simulink model "LP8"  (R2019a)
settings: Solver=FixedStepDiscrete  StartTime=0.0  StopTime=stop_time  RelTol=1e-3
InitFcn:
  | sm_callback_init
StopFcn:
  | sm_callback_stop
undefined symbols (not defined in the file or in its folder): mp
libraries: simulink x3
settings Model: Creator=Ross  LastModifiedBy=Ross
settings DataIOCC: ReturnWorkspaceOutputs=off
settings OptimizationCC: BlockReduction=off  ConditionallyExecuteInputs=off  DefaultParameterBehavior=Inlined
settings DebuggingCC: ReadBeforeWriteMsg=DisableAll  WriteAfterWriteMsg=DisableAll  WriteAfterReadMsg=DisableAll  AlgebraicLoopMsg=error  MultiTaskDSMMsg=none  SingleTaskRateTransMsg=error  PregeneratedLibrarySubsystemCodeDiagnostic=none  ArithmeticOperatorsInVariantConditions=warning
settings HardwareCC: ProdBitPerPointer=32  ProdBitPerSizeT=32  ProdBitPerPtrDiffT=32  ProdLargestAtomicFloat=None  ProdIntDivRoundTo=Undefined  ProdEndianess=Unspecified  ProdWordSize=32  ProdHWDeviceType=ASIC/FPGA->ASIC/FPGA  TargetBitPerPointer=64  TargetBitPerSizeT=64  TargetBitPerPtrDiffT=64  TargetLongLongMode=on  TargetIntDivRoundTo=Zero  TargetEndianess=LittleEndian  TargetWordSize=64  TargetHWDeviceType=Custom Processor->MATLAB Host Computer  ProdEqTarget=off
settings ModelReferenceCC: UpdateModelReferenceTargets=IfOutOfDate
settings SFSimCC: SFSimEcho=off  SimUseLocalCustomCode=off
settings RTWCC: RTWUseLocalCustomCode=off

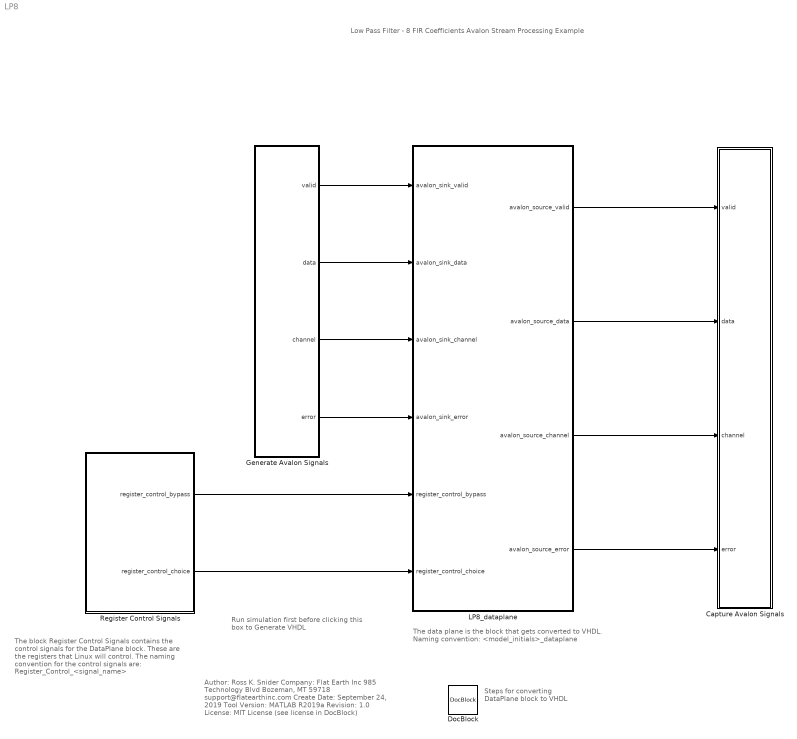
== system LP8 ==
  note: The data plane is the block that gets converted to VHDL. Naming convention: <model_initials>_dataplane
  note: Author:          Ross K. Snider
      | Company:     Flat Earth Inc
      |                       985 Technology Blvd
      |                       Bozeman, MT 59718
      |                       support@flatearthinc.com
      | Create Date:  September 24, 2019
      | Tool Version:  MATLAB R2019a
      | Revision:        1.0
      | License:          MIT License (see license in DocBlock)
  note: Steps for converting
      | DataPlane block
      | to VHDL
  note: Low Pass Filter - 8 FIR Coefficients
      | Avalon Stream Processing Example
  note: Run simulation first
      | before clicking this box to
      | Generate VHDL
  note: The block Register Control Signals contains
      | the control signals for the DataPlane block.
      | These are the registers that Linux will control.
      | The naming convention for the control
      | signals are:  Register_Control_<signal_name>
  Capture Avalon Signals : Subsystem
  DocBlock : simulink/Model-Wide Utilities/DocBlock  DocumentType=HTML
  Generate Avalon Signals : Subsystem
  LP8_dataplane : Subsystem  TreatAsAtomicUnit=on
  Register Control Signals : Subsystem
  wires:
  Generate Avalon Signals/2(data) -> LP8_dataplane/2(avalon_sink_data)
  Generate Avalon Signals/1(valid) -> LP8_dataplane/1(avalon_sink_valid)
  Generate Avalon Signals/3(channel) -> LP8_dataplane/3(avalon_sink_channel)
  Generate Avalon Signals/4(error) -> LP8_dataplane/4(avalon_sink_error)
  LP8_dataplane/2(avalon_source_data) -> Capture Avalon Signals/2(data)
  LP8_dataplane/1(avalon_source_valid) -> Capture Avalon Signals/1(valid)
  LP8_dataplane/3(avalon_source_channel) -> Capture Avalon Signals/3(channel)
  LP8_dataplane/4(avalon_source_error) -> Capture Avalon Signals/4(error)
  Register Control Signals/2(register_control_choice) -> LP8_dataplane/6(register_control_choice)
  Register Control Signals/1(register_control_bypass) -> LP8_dataplane/5(register_control_bypass)

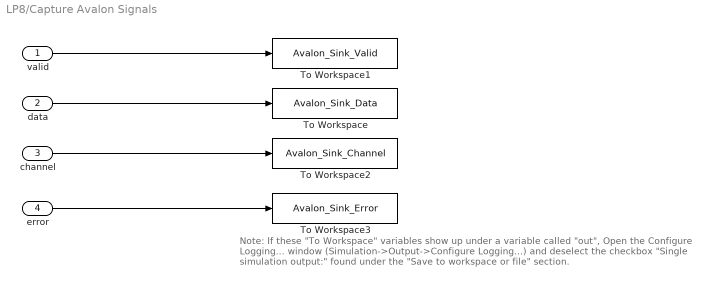
== system LP8/Capture Avalon Signals ==
  note: Note:  If these "To Workspace" variables show up under a variable called "out",
      | Open the Configure Logging... window (Simulation->Output->Configure Logging...)
      | and deselect the checkbox "Single simulation output:" found under the "Save to workspace or file" section.
  valid : Inport
  data : Inport  Port=2
  channel : Inport  Port=3
  error : Inport  Port=4
  To Workspace : ToWorkspace  VariableName=Avalon_Sink_Data  SaveFormat=Timeseries  SampleTime=-1
  To Workspace1 : ToWorkspace  VariableName=Avalon_Sink_Valid  SaveFormat=Timeseries  SampleTime=-1
  To Workspace2 : ToWorkspace  VariableName=Avalon_Sink_Channel  SaveFormat=Timeseries  SampleTime=-1
  To Workspace3 : ToWorkspace  VariableName=Avalon_Sink_Error  SaveFormat=Timeseries  SampleTime=-1
  wires:
  data/1 -> To Workspace/1
  valid/1 -> To Workspace1/1
  error/1 -> To Workspace3/1
  channel/1 -> To Workspace2/1

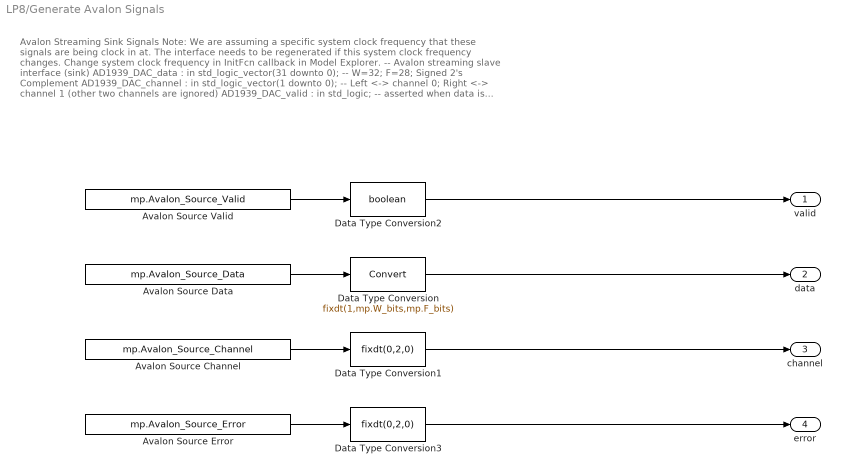
== system LP8/Generate Avalon Signals ==
  note: Avalon Streaming Sink Signals
      | Note: We are assuming a specific system clock frequency that these signals are being clock in at.
      | The interface needs to be regenerated if this system clock frequency changes. Change system clock frequency in InitFcn callback in Model Explorer.
      |
      | -- Avalon streaming slave interface (sink)
      | AD1939_DAC_data : in std_logic_vector(31 downto 0); -- W=32; F=28; Signed 2's Complement
      | AD1939_DAC_channel : in std_logic_vector(1 downto 0); -- Left <-> channel 0; Right <-> channel 1 (other two channels are ignored)
      | AD1939_DAC_valid : in std_logic; -- asserted when data is valid
      | AD1939_DAC_error : in std_logic_vector(1 downto 0) -- error channel is ignored, assumed to be error free at this point
      |
      | For more information on the data-channel-valid protocol, s ee chapter 5 in Intel's Avalon Interfaced Specification (p. 40) at https://www.intel.com/content/dam/www/programmable/us/en/pdfs/literature/manual/mnl_avalon_spec.pdf
  Avalon Source Channel : FromWorkspace  VariableName=mp.Avalon_Source_Channel  OutDataTypeStr=double  SampleTime=mp.Ts_system
  "Avalon Source Data " : FromWorkspace  VariableName=mp.Avalon_Source_Data  OutDataTypeStr=double  SampleTime=mp.Ts_system
  Avalon Source Error : FromWorkspace  VariableName=mp.Avalon_Source_Error  OutDataTypeStr=double  SampleTime=mp.Ts_system
  Avalon Source Valid : FromWorkspace  VariableName=mp.Avalon_Source_Valid  OutDataTypeStr=double  SampleTime=mp.Ts_system
  Data Type Conversion : DataTypeConversion  OutDataTypeStr=fixdt(1,mp.W_bits,mp.F_bits)
  Data Type Conversion1 : DataTypeConversion  OutDataTypeStr=fixdt(0,2,0)
  Data Type Conversion2 : DataTypeConversion  OutDataTypeStr=boolean
  Data Type Conversion3 : DataTypeConversion  OutDataTypeStr=fixdt(0,2,0)
  valid : Outport
  data : Outport  Port=2
  channel : Outport  Port=3
  error : Outport  Port=4
  wires:
  Data Type Conversion1/1 -> channel/1
  Data Type Conversion2/1 -> valid/1
  Avalon Source Error/1 -> Data Type Conversion3/1
  Data Type Conversion/1 -> data/1
  Avalon Source Valid/1 -> Data Type Conversion2/1
  Data Type Conversion3/1 -> error/1
  Avalon Source Channel/1 -> Data Type Conversion1/1
  "Avalon Source Data "/1 -> Data Type Conversion/1

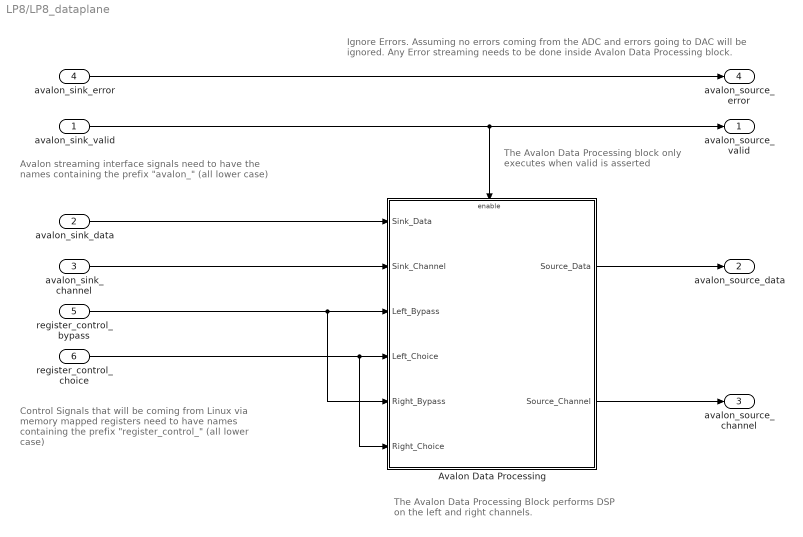
== system LP8/LP8_dataplane ==
  note: Control Signals that will be coming from Linux via
      | memory mapped registers need to have names
      | containing the prefix "register_control_"
      | (all lower case)
  note: The Avalon Data Processing Block
      | performs DSP on the left and right channels.
  note: The Avalon Data Processing block
      | only executes when valid is asserted
  note: Ignore Errors.
      | Assuming no errors coming from the ADC and errors going to DAC will be ignored.
      | Any Error streaming needs to be done inside Avalon Data Processing block.
  note: Avalon streaming interface signals need to have the
      | names containing the prefix "avalon_"
      | (all lower case)
  avalon_sink_valid : Inport
  avalon_sink_data : Inport  Port=2
  avalon_sink_channel : Inport  Port=3
  avalon_sink_error : Inport  Port=4
  register_control_bypass : Inport  Port=5
  register_control_choice : Inport  Port=6
  Avalon Data Processing : Subsystem  TreatAsAtomicUnit=on
  avalon_source_valid : Outport
  avalon_source_data : Outport  Port=2
  avalon_source_channel : Outport  Port=3
  avalon_source_error : Outport  Port=4
  wires:
  avalon_sink_channel/1 -> Avalon Data Processing/2(Sink_Channel)
  avalon_sink_error/1 -> avalon_source_error/1
  Avalon Data Processing/1(Source_Data) -> avalon_source_data/1
  avalon_sink_valid/1 -> avalon_source_valid/1, Avalon Data Processing/Enable
  avalon_sink_data/1 -> Avalon Data Processing/1(Sink_Data)
  Avalon Data Processing/2(Source_Channel) -> avalon_source_channel/1
  register_control_bypass/1 -> Avalon Data Processing/5(Right_Bypass), Avalon Data Processing/3(Left_Bypass)
  register_control_choice/1 -> Avalon Data Processing/6(Right_Choice), Avalon Data Processing/4(Left_Choice)

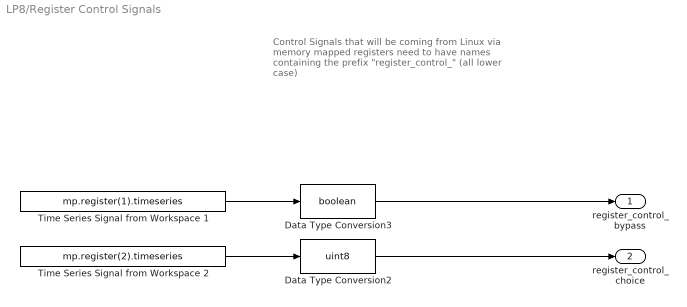
== system LP8/Register Control Signals ==
  note: Control Signals that will be coming from Linux via
      | memory mapped registers need to have names
      | containing the prefix "register_control_"
      | (all lower case)
  Data Type Conversion2 : DataTypeConversion  OutDataTypeStr=uint8
  Data Type Conversion3 : DataTypeConversion  OutDataTypeStr=boolean
  Time Series Signal from Workspace 1 : FromWorkspace  VariableName=mp.register(1).timeseries  OutDataTypeStr=double  SampleTime=mp.Ts_system
  Time Series Signal from Workspace 2 : FromWorkspace  VariableName=mp.register(2).timeseries  OutDataTypeStr=double  SampleTime=mp.Ts_system
  register_control_bypass : Outport
  register_control_choice : Outport  Port=2
  wires:
  Time Series Signal from Workspace 2/1 -> Data Type Conversion2/1
  Data Type Conversion2/1 -> register_control_choice/1
  Time Series Signal from Workspace 1/1 -> Data Type Conversion3/1
  Data Type Conversion3/1 -> register_control_bypass/1

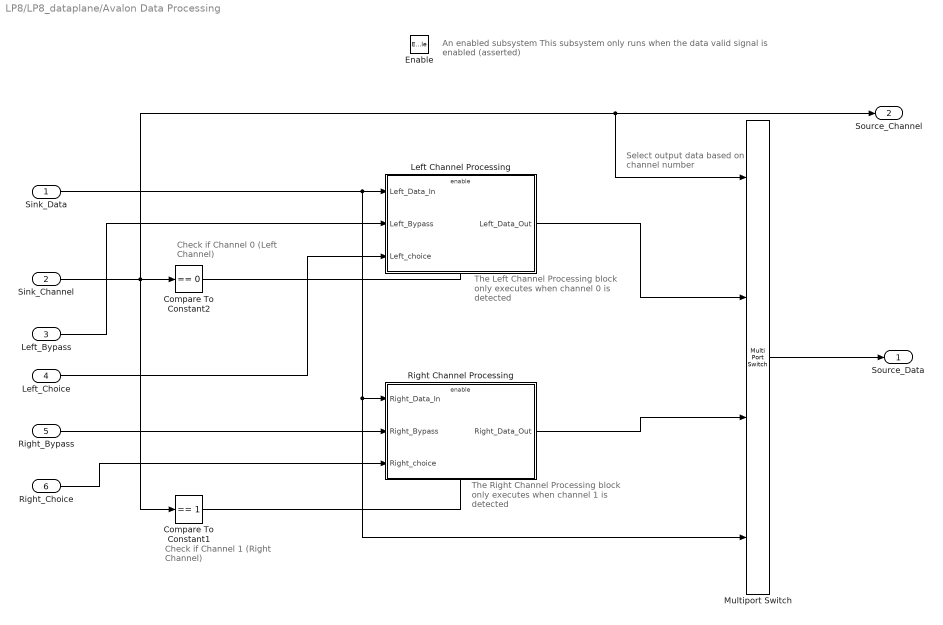
== system LP8/LP8_dataplane/Avalon Data Processing ==
  note: Select output data
      | based on channel number
  note: Check if Channel 0
      | (Left Channel)
  note: The Left Channel Processing block
      | only executes when channel 0
      | is detected
  note: The Right Channel Processing block
      | only executes when channel 1
      | is detected
  note: Check if Channel 1
      | (Right Channel)
  note: An enabled subsystem
      | This subsystem only runs when the data valid signal is enabled (asserted)
  Sink_Data : Inport
  Sink_Channel : Inport  Port=2
  Left_Bypass : Inport  Port=3
  Left_Choice : Inport  Port=4
  Right_Bypass : Inport  Port=5
  Right_Choice : Inport  Port=6
  Enable : EnablePort
  Compare To Constant1 : simulink/Logic and Bit Operations/Compare To Constant  relop===  const=1  OutDataTypeStr=boolean
  Compare To Constant2 : simulink/Logic and Bit Operations/Compare To Constant  relop===  const=0  OutDataTypeStr=boolean
  Left Channel Processing : Subsystem  TreatAsAtomicUnit=on
  Multiport Switch : MultiPortSwitch  DataPortOrder=Zero-based contiguous  zeroidx=on
  Right Channel Processing : Subsystem  TreatAsAtomicUnit=on
  Source_Data : Outport  InitialOutput=0
  Source_Channel : Outport  Port=2  InitialOutput=0
  wires:
  Sink_Channel/1 -> Source_Channel/1, Multiport Switch/1, Compare To Constant1/1, Compare To Constant2/1
  Compare To Constant2/1 -> Left Channel Processing/Enable
  Compare To Constant1/1 -> Right Channel Processing/Enable
  Sink_Data/1 -> Multiport Switch/4, Right Channel Processing/1(Right_Data_In), Left Channel Processing/1(Left_Data_In)
  Left Channel Processing/1("Left_Data_Out ") -> Multiport Switch/2
  Right Channel Processing/1("Right_Data_Out ") -> Multiport Switch/3
  Multiport Switch/1 -> Source_Data/1
  Left_Bypass/1 -> Left Channel Processing/2(Left_Bypass)
  Right_Bypass/1 -> Right Channel Processing/2(Right_Bypass)
  Left_Choice/1 -> Left Channel Processing/3(Left_choice)
  Right_Choice/1 -> Right Channel Processing/3(Right_choice)

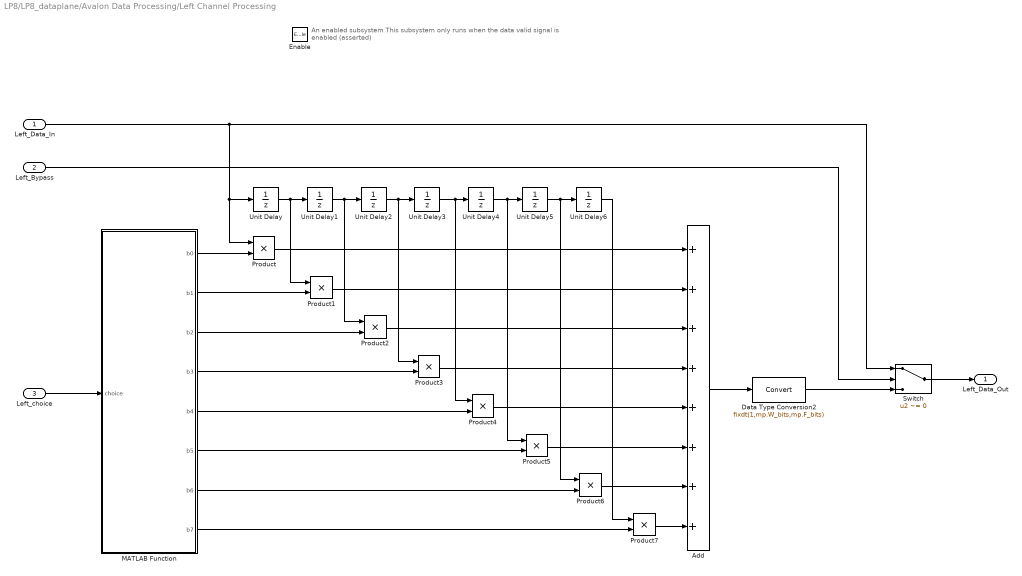
== system LP8/LP8_dataplane/Avalon Data Processing/Left Channel Processing ==
  note: An enabled subsystem
      | This subsystem only runs when the data valid signal is enabled (asserted)
  Left_Data_In : Inport
  Left_Bypass : Inport  Port=2
  Left_choice : Inport  Port=3
  Enable : EnablePort
  Add : Sum  Inputs=++++++++
  Data Type Conversion2 : DataTypeConversion  OutDataTypeStr=fixdt(1,mp.W_bits,mp.F_bits)
  MATLAB Function : MATLAB Function  TreatAsAtomicUnit=on
  Product{,1..7} (8 alike) : Product
  Switch : Switch  Criteria=u2 ~= 0
  Unit Delay{,1..6} (7 alike) : UnitDelay  SampleTime=-1  HasFrameUpgradeWarning=on
  "Left_Data_Out " : Outport  InitialOutput=0
  wires:
  Left_Data_In/1 -> Product/1, Unit Delay/1, Switch/1
  Data Type Conversion2/1 -> Switch/3
  Switch/1 -> "Left_Data_Out "/1
  Left_Bypass/1 -> Switch/2
  Unit Delay/1 -> Product1/1, Unit Delay1/1
  Unit Delay1/1 -> Product2/1, Unit Delay2/1
  Unit Delay2/1 -> Product3/1, Unit Delay3/1
  Unit Delay3/1 -> Product4/1, Unit Delay4/1
  Unit Delay4/1 -> Product5/1, Unit Delay5/1
  Unit Delay5/1 -> Product6/1, Unit Delay6/1
  Unit Delay6/1 -> Product7/1
  Product/1 -> Add/1
  Product1/1 -> Add/2
  Product2/1 -> Add/3
  Product3/1 -> Add/4
  Product4/1 -> Add/5
  Product5/1 -> Add/6
  Product6/1 -> Add/7
  Product7/1 -> Add/8
  Add/1 -> Data Type Conversion2/1
  MATLAB Function/1(b0) -> Product/2
  MATLAB Function/8(b7) -> Product7/2
  MATLAB Function/2(b1) -> Product1/2
  MATLAB Function/3(b2) -> Product2/2
  MATLAB Function/4(b3) -> Product3/2
  MATLAB Function/5(b4) -> Product4/2
  MATLAB Function/6(b5) -> Product5/2
  MATLAB Function/7(b6) -> Product6/2
  Left_choice/1 -> MATLAB Function/1(choice)

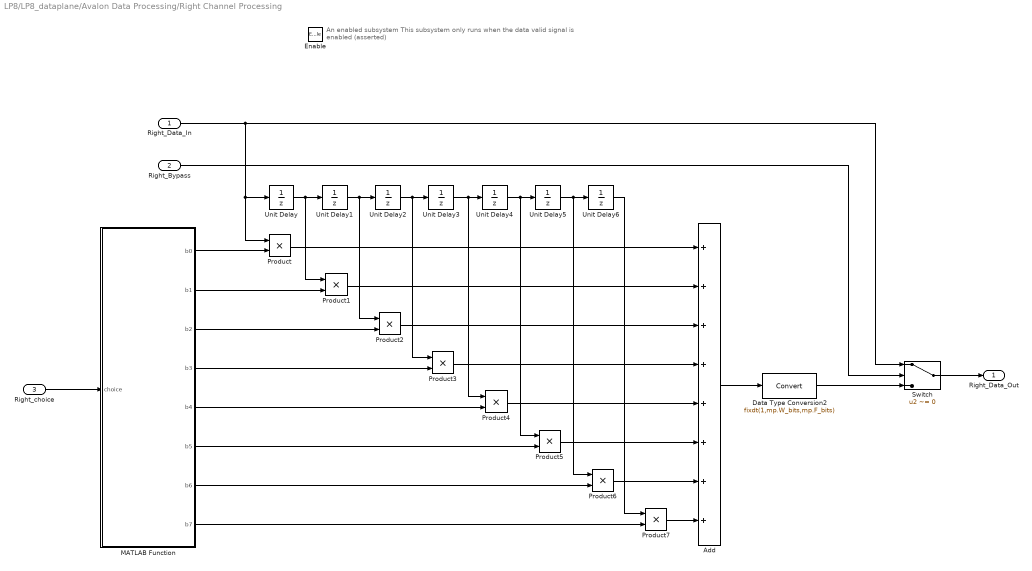
== system LP8/LP8_dataplane/Avalon Data Processing/Right Channel Processing ==
  note: An enabled subsystem
      | This subsystem only runs when the data valid signal is enabled (asserted)
  Right_Data_In : Inport
  Right_Bypass : Inport  Port=2
  Right_choice : Inport  Port=3
  Enable : EnablePort
  Add : Sum  Inputs=++++++++
  Data Type Conversion2 : DataTypeConversion  OutDataTypeStr=fixdt(1,mp.W_bits,mp.F_bits)
  MATLAB Function : MATLAB Function  TreatAsAtomicUnit=on
  Product{,1..7} (8 alike) : Product
  Switch : Switch  Criteria=u2 ~= 0
  Unit Delay{,1..6} (7 alike) : UnitDelay  SampleTime=-1  HasFrameUpgradeWarning=on
  "Right_Data_Out " : Outport  InitialOutput=0
  wires:
  Right_Data_In/1 -> Product/1, Unit Delay/1, Switch/1
  Data Type Conversion2/1 -> Switch/3
  Switch/1 -> "Right_Data_Out "/1
  Right_Bypass/1 -> Switch/2
  Unit Delay/1 -> Product1/1, Unit Delay1/1
  Unit Delay1/1 -> Product2/1, Unit Delay2/1
  Unit Delay2/1 -> Product3/1, Unit Delay3/1
  Unit Delay3/1 -> Product4/1, Unit Delay4/1
  Unit Delay4/1 -> Product5/1, Unit Delay5/1
  Unit Delay5/1 -> Product6/1, Unit Delay6/1
  Unit Delay6/1 -> Product7/1
  Product/1 -> Add/1
  Product1/1 -> Add/2
  Product2/1 -> Add/3
  Product3/1 -> Add/4
  Product4/1 -> Add/5
  Product5/1 -> Add/6
  Product6/1 -> Add/7
  Product7/1 -> Add/8
  Add/1 -> Data Type Conversion2/1
  MATLAB Function/1(b0) -> Product/2
  MATLAB Function/8(b7) -> Product7/2
  MATLAB Function/2(b1) -> Product1/2
  MATLAB Function/3(b2) -> Product2/2
  MATLAB Function/4(b3) -> Product3/2
  MATLAB Function/5(b4) -> Product4/2
  MATLAB Function/6(b5) -> Product5/2
  MATLAB Function/7(b6) -> Product6/2
  Right_choice/1 -> MATLAB Function/1(choice)

== matlab function LP8/LP8_dataplane/Avalon Data Processing/Right Channel Processing/MATLAB Function ==
  data: choice input; b0 output; b1 output; b2 output; b3 output; b4 output; b5 output; b6 output; b7 output
function [b0, b1, b2, b3, b4, b5, b6, b7] = get_coefficients(choice)
switch(choice)
    case 1
        b0 = fi(0.0181749831525104474372334096,0,32,28);
        b1 = fi(0.0487938812952927875032926863,0,32,28);
        b2 = fi(0.1227231904517332439219501339,0,32,28);
        b3 = fi(0.1966623798866671546381468261,0,32,28);
        b4 = fi(0.2272911304275925525875123867,0,32,28);
        b5 = fi(0.1966623798866671546381468261,0,32,28);
        b6 = fi(0.1227231904517332439219501339,0,32,28);
        b7 = fi(0.0487938812952927875032926863,0,32,28);
    case 2
        b0 = fi(0.0181679661831235239599635634,0,32,28);
        b1 = fi(0.0487850597667578433913604385,0,32,28);
        b2 = fi(0.1227189978688955629415602289,0,32,28);
        b3 = fi(0.1966729627794475687707631550,0,32,28);
        b4 = fi(0.2273100268035510573838564596,0,32,28);
        b5 = fi(0.1966729627794475687707631550,0,32,28);
        b6 = fi(0.1227189978688955629415602289,0,32,28);
        b7 = fi(0.0487850597667578433913604385,0,32,28);
    case 3
        b0 = fi(0.0181537475815499449449674785,0,32,28);
        b1 = fi(0.0487671806703944485383850349,0,32,28);
        b2 = fi(0.1227104972644888769561788422,0,32,28);
        b3 = fi(0.1966944108526903489675419223,0,32,28);
        b4 = fi(0.2273483272617527195524900208,0,32,28);
        b5 = fi(0.1966944108526903489675419223,0,32,28);
        b6 = fi(0.1227104972644888769561788422,0,32,28);
        b7 = fi(0.0487671806703944485383850349,0,32,28);
    case 4
        b0 = fi(0.0181249427844423181832578251,0,32,28);
        b1 = fi(0.0487309442828232769473473240,0,32,28);
        b2 = fi(0.1226932553174884116264919953,0,32,28);
        b3 = fi(0.1967378770332015858190999325,0,32,28);
        b4 = fi(0.2274259611640887801531363266,0,32,28);
        b5 = fi(0.1967378770332015858190999325,0,32,28);
        b6 = fi(0.1226932553174884116264919953,0,32,28);
        b7 = fi(0.0487309442828232769473473240,0,32,28);
    case 5
        b0 = fi(0.0180666155875539510833327483,0,32,28);
        b1 = fi(0.0486575031751405109869956789,0,32,28);
        b2 = fi(0.1226582556935295054145740323,0,32,28);
        b3 = fi(0.1968259560791854323458238696,0,32,28);
        b4 = fi(0.2275833389291813668720010355,0,32,28);
        b5 = fi(0.1968259560791854323458238696,0,32,28);
        b6 = fi(0.1226582556935295054145740323,0,32,28);
        b7 = fi(0.0486575031751405109869956789,0,32,28);
    case 6
        b0 = fi(0.0179486194922491119896346135,0,32,28);
        b1 = fi(0.0485086621264032222256012972,0,32,28);
        b2 = fi(0.1225870969701776391769243446,0,32,28);
        b3 = fi(0.1970044025265542397828966159,0,32,28);
        b4 = fi(0.2279024377692315250776289304,0,32,28);
        b5 = fi(0.1970044025265542397828966159,0,32,28);
        b6 = fi(0.1225870969701776391769243446,0,32,28);
        b7 = fi(0.0485086621264032222256012972,0,32,28);
    case 7
        b0 = fi(0.0177103714480851583135123661,0,32,28);
        b1 = fi(0.0482070272552556286504987781,0,32,28);
        b2 = fi(0.1224419605994097881573878794,0,32,28);
        b3 = fi(0.1973657849491358140525676390,0,32,28);
        b4 = fi(0.2285497114962272979798996175,0,32,28);
        b5 = fi(0.1973657849491358140525676390,0,32,28);
        b6 = fi(0.1224419605994097881573878794,0,32,28);
        b7 = fi(0.0482070272552556286504987781,0,32,28);
    case 8
        b0 = fi(0.0172312108373964441299097672,0,32,28);
        b1 = fi(0.0475958332873485656655532239,0,32,28);
        b2 = fi(0.1221440501723489169272340860,0,32,28);
        b3 = fi(0.1980970246956992864006963373,0,32,28);
        b4 = fi(0.2298637620144136362032583065,0,32,28);
        b5 = fi(0.1980970246956992864006963373,0,32,28);
        b6 = fi(0.1221440501723489169272340860,0,32,28);
        b7 = fi(0.0475958332873485656655532239,0,32,28);
    case 9
        b0 = fi(0.0162753544931512200699685877,0,32,28);
        b1 = fi(0.0463578756874775746443795299,0,32,28);
        b2 = fi(0.1215248623454721760284158449,0,32,28);
        b3 = fi(0.1995739951288263425155378172,0,32,28);
        b4 = fi(0.2325358246901454983834867107,0,32,28);
        b5 = fi(0.1995739951288263425155378172,0,32,28);
        b6 = fi(0.1215248623454721760284158449,0,32,28);
        b7 = fi(0.0463578756874775746443795299,0,32,28);
    case 10
        b0 = fi(0.0144011579357415601260195004,0,32,28);
        b1 = fi(0.0438535301436539654007518152,0,32,28);
        b2 = fi(0.1202069083649044134443073517,0,32,28);
        b3 = fi(0.2025452706676268699315102140,0,32,28);
        b4 = fi(0.2379862657761463440309057660,0,32,28);
        b5 = fi(0.2025452706676268699315102140,0,32,28);
        b6 = fi(0.1202069083649044134443073517,0,32,28);
        b7 = fi(0.0438535301436539654007518152,0,32,28);
    case 11
        b0 = fi(0.0108635903091277956356019985,0,32,28);
        b1 = fi(0.0388092965418767935070754049,0,32,28);
        b2 = fi(0.1172793972292393016587652710,0,32,28);
        b3 = fi(0.2084652871331992840531199818,0,32,28);
        b4 = fi(0.2491648575731136017186173603,0,32,28);
        b5 = fi(0.2084652871331992840531199818,0,32,28);
        b6 = fi(0.1172793972292393016587652710,0,32,28);
        b7 = fi(0.0388092965418767935070754049,0,32,28);
    case 12
        b0 = fi(0.0047698697834522539584778400,0,32,28);
        b1 = fi(0.0288154849920489834758097203,0,32,28);
        b2 = fi(0.1103238404973209407788914405,0,32,28);
        b3 = fi(0.2199570517909645861465151029,0,32,28);
        b4 = fi(0.2722675058724263186249459068,0,32,28);
        b5 = fi(0.2199570517909645861465151029,0,32,28);
        b6 = fi(0.1103238404973209407788914405,0,32,28);
        b7 = fi(0.0288154849920489834758097203,0,32,28);
    case 13
        b0 = fi(-0.0033065810459098161563917806,0,32,28);
        b1 = fi(0.0102885652143332850111390186,0,32,28);
        b2 = fi(0.0924417634408608857032874084,0,32,28);
        b3 = fi(0.2405174387604489816272490543,0,32,28);
        b4 = fi(0.3201176272605333328336030263,0,32,28);
        b5 = fi(0.2405174387604489816272490543,0,32,28);
        b6 = fi(0.0924417634408608857032874084,0,32,28);
        b7 = fi(0.0102885652143332850111390186,0,32,28);
    case 14
        b0 = fi(-0.0057790702811202120450784214,0,32,28);
        b1 = fi(-0.0154110030477560781131396439,0,32,28);
        b2 = fi(0.0459887543145310606629294625,0,32,28);
        b3 = fi(0.2674984498139851840647907011,0,32,28);
        b4 = fi(0.4154057384007200925957192794,0,32,28);
        b5 = fi(0.2674984498139851840647907011,0,32,28);
        b6 = fi(0.0459887543145310606629294625,0,32,28);
        b7 = fi(-0.0154110030477560781131396439,0,32,28);
    case 15
        b0 = fi(0.0055463527953608787735007013,0,32,28);
        b1 = fi(-0.0156715004641111363414829327,0,32,28);
        b2 = fi(-0.0435518863745886150584674112,0,32,28);
        b3 = fi(0.2634025670382789674484058651,0,32,28);
        b4 = fi(0.5805489340101198658672387864,0,32,28);
        b5 = fi(0.2634025670382789674484058651,0,32,28);
        b6 = fi(-0.0435518863745886150584674112,0,32,28);
        b7 = fi(-0.0156715004641111363414829327,0,32,28);
    case 16
        b0 = fi(-0.0055441199344672701873615317,0,32,28);
        b1 = fi(0.0229110630161322506581633718,0,32,28);
        b2 = fi(-0.0748456191153083483236230222,0,32,28);
        b3 = fi(0.1384819588513515609129456152,0,32,28);
        b4 = fi(0.8379934343645835115310660512,0,32,28);
        b5 = fi(0.1384819588513515609129456152,0,32,28);
        b6 = fi(-0.0748456191153083483236230222,0,32,28);
        b7 = fi(0.0229110630161322506581633718,0,32,28);
    otherwise
        b0 = fi(-0.0055441199344672701873615317,0,32,28);
        b1 = fi(0.0229110630161322506581633718,0,32,28);
        b2 = fi(-0.0748456191153083483236230222,0,32,28);
        b3 = fi(0.1384819588513515609129456152,0,32,28);
        b4 = fi(0.8379934343645835115310660512,0,32,28);
        b5 = fi(0.1384819588513515609129456152,0,32,28);
        b6 = fi(-0.0748456191153083483236230222,0,32,28);
        b7 = fi(0.0229110630161322506581633718,0,32,28);        
end

== matlab function LP8/LP8_dataplane/Avalon Data Processing/Left Channel Processing/MATLAB Function ==
  data: choice input; b0 output; b1 output; b2 output; b3 output; b4 output; b5 output; b6 output; b7 output
function [b0, b1, b2, b3, b4, b5, b6, b7] = get_coefficients(choice)
switch(choice)
    case 1
        b0 = fi(0.0181749831525104474372334096,0,32,28);
        b1 = fi(0.0487938812952927875032926863,0,32,28);
        b2 = fi(0.1227231904517332439219501339,0,32,28);
        b3 = fi(0.1966623798866671546381468261,0,32,28);
        b4 = fi(0.2272911304275925525875123867,0,32,28);
        b5 = fi(0.1966623798866671546381468261,0,32,28);
        b6 = fi(0.1227231904517332439219501339,0,32,28);
        b7 = fi(0.0487938812952927875032926863,0,32,28);
    case 2
        b0 = fi(0.0181679661831235239599635634,0,32,28);
        b1 = fi(0.0487850597667578433913604385,0,32,28);
        b2 = fi(0.1227189978688955629415602289,0,32,28);
        b3 = fi(0.1966729627794475687707631550,0,32,28);
        b4 = fi(0.2273100268035510573838564596,0,32,28);
        b5 = fi(0.1966729627794475687707631550,0,32,28);
        b6 = fi(0.1227189978688955629415602289,0,32,28);
        b7 = fi(0.0487850597667578433913604385,0,32,28);
    case 3
        b0 = fi(0.0181537475815499449449674785,0,32,28);
        b1 = fi(0.0487671806703944485383850349,0,32,28);
        b2 = fi(0.1227104972644888769561788422,0,32,28);
        b3 = fi(0.1966944108526903489675419223,0,32,28);
        b4 = fi(0.2273483272617527195524900208,0,32,28);
        b5 = fi(0.1966944108526903489675419223,0,32,28);
        b6 = fi(0.1227104972644888769561788422,0,32,28);
        b7 = fi(0.0487671806703944485383850349,0,32,28);
    case 4
        b0 = fi(0.0181249427844423181832578251,0,32,28);
        b1 = fi(0.0487309442828232769473473240,0,32,28);
        b2 = fi(0.1226932553174884116264919953,0,32,28);
        b3 = fi(0.1967378770332015858190999325,0,32,28);
        b4 = fi(0.2274259611640887801531363266,0,32,28);
        b5 = fi(0.1967378770332015858190999325,0,32,28);
        b6 = fi(0.1226932553174884116264919953,0,32,28);
        b7 = fi(0.0487309442828232769473473240,0,32,28);
    case 5
        b0 = fi(0.0180666155875539510833327483,0,32,28);
        b1 = fi(0.0486575031751405109869956789,0,32,28);
        b2 = fi(0.1226582556935295054145740323,0,32,28);
        b3 = fi(0.1968259560791854323458238696,0,32,28);
        b4 = fi(0.2275833389291813668720010355,0,32,28);
        b5 = fi(0.1968259560791854323458238696,0,32,28);
        b6 = fi(0.1226582556935295054145740323,0,32,28);
        b7 = fi(0.0486575031751405109869956789,0,32,28);
    case 6
        b0 = fi(0.0179486194922491119896346135,0,32,28);
        b1 = fi(0.0485086621264032222256012972,0,32,28);
        b2 = fi(0.1225870969701776391769243446,0,32,28);
        b3 = fi(0.1970044025265542397828966159,0,32,28);
        b4 = fi(0.2279024377692315250776289304,0,32,28);
        b5 = fi(0.1970044025265542397828966159,0,32,28);
        b6 = fi(0.1225870969701776391769243446,0,32,28);
        b7 = fi(0.0485086621264032222256012972,0,32,28);
    case 7
        b0 = fi(0.0177103714480851583135123661,0,32,28);
        b1 = fi(0.0482070272552556286504987781,0,32,28);
        b2 = fi(0.1224419605994097881573878794,0,32,28);
        b3 = fi(0.1973657849491358140525676390,0,32,28);
        b4 = fi(0.2285497114962272979798996175,0,32,28);
        b5 = fi(0.1973657849491358140525676390,0,32,28);
        b6 = fi(0.1224419605994097881573878794,0,32,28);
        b7 = fi(0.0482070272552556286504987781,0,32,28);
    case 8
        b0 = fi(0.0172312108373964441299097672,0,32,28);
        b1 = fi(0.0475958332873485656655532239,0,32,28);
        b2 = fi(0.1221440501723489169272340860,0,32,28);
        b3 = fi(0.1980970246956992864006963373,0,32,28);
        b4 = fi(0.2298637620144136362032583065,0,32,28);
        b5 = fi(0.1980970246956992864006963373,0,32,28);
        b6 = fi(0.1221440501723489169272340860,0,32,28);
        b7 = fi(0.0475958332873485656655532239,0,32,28);
    case 9
        b0 = fi(0.0162753544931512200699685877,0,32,28);
        b1 = fi(0.0463578756874775746443795299,0,32,28);
        b2 = fi(0.1215248623454721760284158449,0,32,28);
        b3 = fi(0.1995739951288263425155378172,0,32,28);
        b4 = fi(0.2325358246901454983834867107,0,32,28);
        b5 = fi(0.1995739951288263425155378172,0,32,28);
        b6 = fi(0.1215248623454721760284158449,0,32,28);
        b7 = fi(0.0463578756874775746443795299,0,32,28);
    case 10
        b0 = fi(0.0144011579357415601260195004,0,32,28);
        b1 = fi(0.0438535301436539654007518152,0,32,28);
        b2 = fi(0.1202069083649044134443073517,0,32,28);
        b3 = fi(0.2025452706676268699315102140,0,32,28);
        b4 = fi(0.2379862657761463440309057660,0,32,28);
        b5 = fi(0.2025452706676268699315102140,0,32,28);
        b6 = fi(0.1202069083649044134443073517,0,32,28);
        b7 = fi(0.0438535301436539654007518152,0,32,28);
    case 11
        b0 = fi(0.0108635903091277956356019985,0,32,28);
        b1 = fi(0.0388092965418767935070754049,0,32,28);
        b2 = fi(0.1172793972292393016587652710,0,32,28);
        b3 = fi(0.2084652871331992840531199818,0,32,28);
        b4 = fi(0.2491648575731136017186173603,0,32,28);
        b5 = fi(0.2084652871331992840531199818,0,32,28);
        b6 = fi(0.1172793972292393016587652710,0,32,28);
        b7 = fi(0.0388092965418767935070754049,0,32,28);
    case 12
        b0 = fi(0.0047698697834522539584778400,0,32,28);
        b1 = fi(0.0288154849920489834758097203,0,32,28);
        b2 = fi(0.1103238404973209407788914405,0,32,28);
        b3 = fi(0.2199570517909645861465151029,0,32,28);
        b4 = fi(0.2722675058724263186249459068,0,32,28);
        b5 = fi(0.2199570517909645861465151029,0,32,28);
        b6 = fi(0.1103238404973209407788914405,0,32,28);
        b7 = fi(0.0288154849920489834758097203,0,32,28);
    case 13
        b0 = fi(-0.0033065810459098161563917806,0,32,28);
        b1 = fi(0.0102885652143332850111390186,0,32,28);
        b2 = fi(0.0924417634408608857032874084,0,32,28);
        b3 = fi(0.2405174387604489816272490543,0,32,28);
        b4 = fi(0.3201176272605333328336030263,0,32,28);
        b5 = fi(0.2405174387604489816272490543,0,32,28);
        b6 = fi(0.0924417634408608857032874084,0,32,28);
        b7 = fi(0.0102885652143332850111390186,0,32,28);
    case 14
        b0 = fi(-0.0057790702811202120450784214,0,32,28);
        b1 = fi(-0.0154110030477560781131396439,0,32,28);
        b2 = fi(0.0459887543145310606629294625,0,32,28);
        b3 = fi(0.2674984498139851840647907011,0,32,28);
        b4 = fi(0.4154057384007200925957192794,0,32,28);
        b5 = fi(0.2674984498139851840647907011,0,32,28);
        b6 = fi(0.0459887543145310606629294625,0,32,28);
        b7 = fi(-0.0154110030477560781131396439,0,32,28);
    case 15
        b0 = fi(0.0055463527953608787735007013,0,32,28);
        b1 = fi(-0.0156715004641111363414829327,0,32,28);
        b2 = fi(-0.0435518863745886150584674112,0,32,28);
        b3 = fi(0.2634025670382789674484058651,0,32,28);
        b4 = fi(0.5805489340101198658672387864,0,32,28);
        b5 = fi(0.2634025670382789674484058651,0,32,28);
        b6 = fi(-0.0435518863745886150584674112,0,32,28);
        b7 = fi(-0.0156715004641111363414829327,0,32,28);
    case 16
        b0 = fi(-0.0055441199344672701873615317,0,32,28);
        b1 = fi(0.0229110630161322506581633718,0,32,28);
        b2 = fi(-0.0748456191153083483236230222,0,32,28);
        b3 = fi(0.1384819588513515609129456152,0,32,28);
        b4 = fi(0.8379934343645835115310660512,0,32,28);
        b5 = fi(0.1384819588513515609129456152,0,32,28);
        b6 = fi(-0.0748456191153083483236230222,0,32,28);
        b7 = fi(0.0229110630161322506581633718,0,32,28);
    otherwise
        b0 = fi(-0.0055441199344672701873615317,0,32,28);
        b1 = fi(0.0229110630161322506581633718,0,32,28);
        b2 = fi(-0.0748456191153083483236230222,0,32,28);
        b3 = fi(0.1384819588513515609129456152,0,32,28);
        b4 = fi(0.8379934343645835115310660512,0,32,28);
        b5 = fi(0.1384819588513515609129456152,0,32,28);
        b6 = fi(-0.0748456191153083483236230222,0,32,28);
        b7 = fi(0.0229110630161322506581633718,0,32,28);        
end
